simulink model "CDPR_INVERSKINEMATIKK_14_09_23"  (R2022b)
settings: Solver=FixedStepAuto  StartTime=0.0  StopTime=10.0  FixedStep=h  RelTol=1e-3
values from neighbouring files (symbols this model uses):
  a1 = A1 - origin    [CDPR_2R_test.m]    (also in CDPR_2T.m; TEST_INVERSKINEMATIKK.m = [0;1])
  a2 = A2 - origin    [CDPR_2R_test.m]    (also in CDPR_2T.m; TEST_INVERSKINEMATIKK.m = [1;1])
  a3 = A3 - origin    [CDPR_2R_test.m]    (also in CDPR_2T.m; TEST_INVERSKINEMATIKK.m = [0;0])
  a4 = A4 - origin    [CDPR_2R_test.m]    (also in CDPR_2T.m; TEST_INVERSKINEMATIKK.m = [1;0])
  b1 = B1 - body_origin    [CDPR_2R_test.m]    (also in CDPR_2T.m; TEST_INVERSKINEMATIKK.m = [0;L_end/2])
  b2 = B2 - body_origin    [CDPR_2R_test.m]    (also in CDPR_2T.m; TEST_INVERSKINEMATIKK.m = [0;-L_end/2])
  p = [0.5;0.5]    [TEST_INVERSKINEMATIKK.m]
settings Model: Creator=magag  LastModifiedBy=magngrot

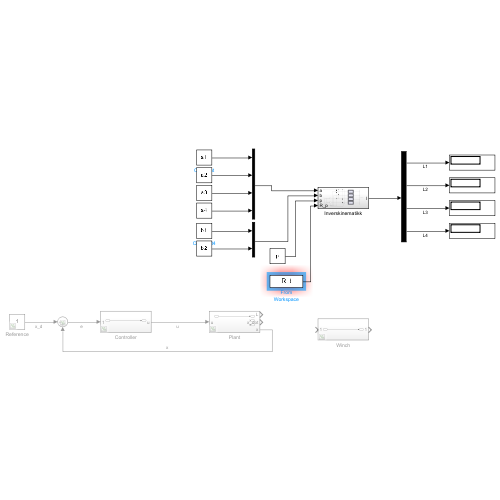
[thumbnail: Simulink's stored preview of the top-level diagram]
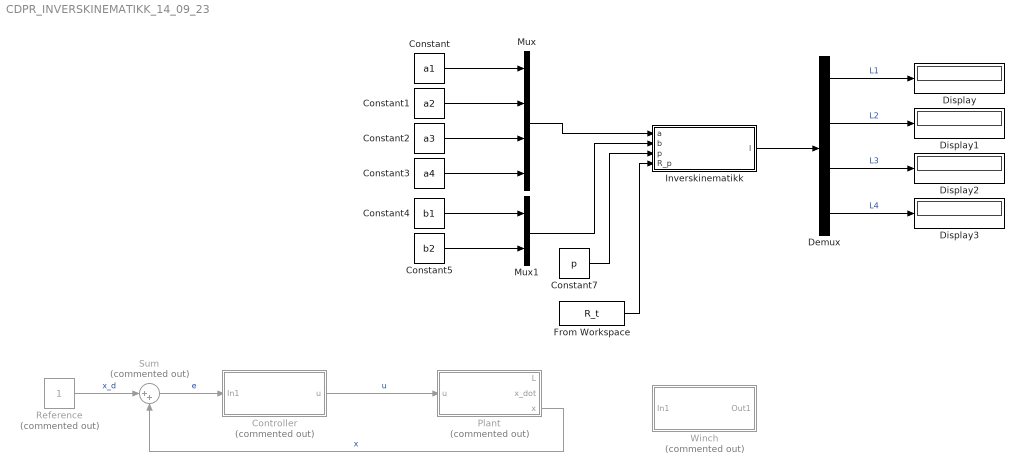
== system CDPR_INVERSKINEMATIKK_14_09_23 ==
  Constant : Constant  Value=a1
  Constant1 : Constant  Value=a2
  Constant2 : Constant  Value=a3
  Constant3 : Constant  Value=a4
  Constant4 : Constant  Value=b1
  Constant5 : Constant  Value=b2
  Constant7 : Constant  Value=p
  Controller : Subsystem  Commented=on
  Demux : Demux
  Display{,1..3} (4 alike) : Display
  From Workspace : FromWorkspace  VariableName=R_t
  Inverskinematikk : Subsystem
  Mux : Mux
  Mux1 : Mux  Inputs=2
  Plant : Subsystem  Commented=on
  Reference : Constant  Commented=on
  Sum : Sum  Commented=on  Inputs=|++
  Winch : Subsystem  Commented=on
  wires:
  Controller/1(u) -> Plant/1(u)  "u"
  Plant/3(x) -> Sum/2  "x"
  Reference/1 -> Sum/1  "x_d"
  Sum/1 -> Controller/1(In1)  "e"
  Constant/1 -> Mux/1
  Constant1/1 -> Mux/2
  Constant2/1 -> Mux/3
  Constant3/1 -> Mux/4
  Mux/1 -> Inverskinematikk/1(a)
  Constant4/1 -> Mux1/1
  Constant5/1 -> Mux1/2
  Mux1/1 -> Inverskinematikk/2(b)
  Inverskinematikk/1(l) -> Demux/1
  Demux/1 -> Display/1  "L1"
  Demux/2 -> Display1/1  "L2"
  Demux/3 -> Display2/1  "L3"
  Demux/4 -> Display3/1  "L4"
  From Workspace/1 -> Inverskinematikk/4(R_p)
  Constant7/1 -> Inverskinematikk/3(p)

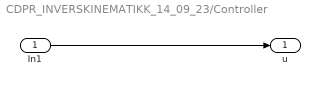
== system CDPR_INVERSKINEMATIKK_14_09_23/Controller ==
  In1 : Inport
  u : Outport
  wires:
  In1/1 -> u/1

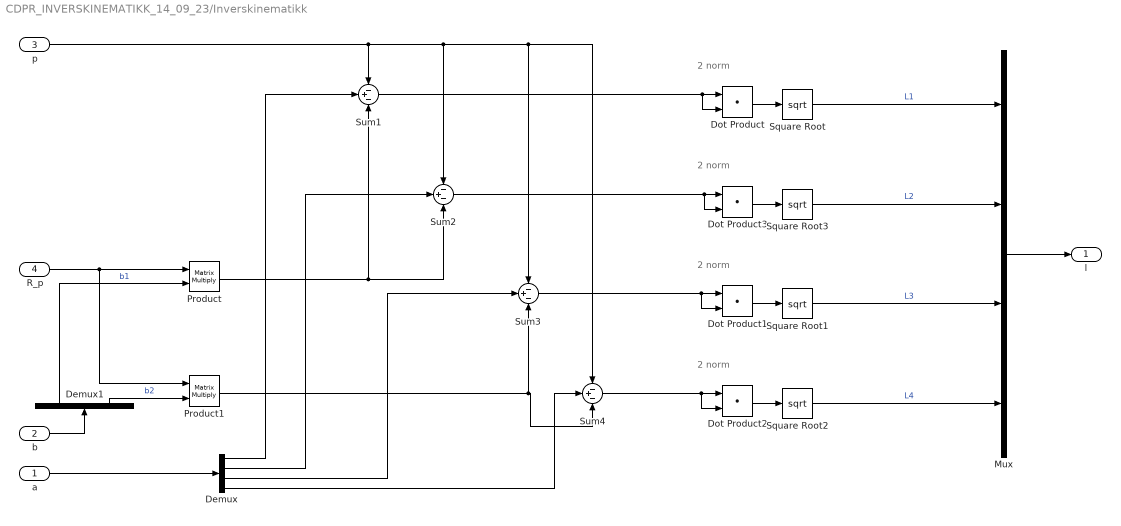
== system CDPR_INVERSKINEMATIKK_14_09_23/Inverskinematikk ==
  note: 2 norm
  note: 2 norm
  note: 2 norm
  note: 2 norm
  a : Inport
  b : Inport  Port=2
  p : Inport  Port=3
  R_p : Inport  Port=4
  Demux : Demux
  Demux1 : Demux  Outputs=2
  Dot Product{,1..3} (4 alike) : DotProduct  OutDataTypeStr=Inherit: Inherit via internal rule
  Mux : Mux
  Product : Product  Multiplication=Matrix(*)
  Product1 : Product  Multiplication=Matrix(*)
  Square Root{,1..3} (4 alike) : Sqrt
  Sum{1..4} (4 alike) : Sum  Inputs=-+-
  l : Outport
  wires:
  R_p/1 -> Product/1, Product1/1
  Dot Product/1 -> Square Root/1
  a/1 -> Demux/1
  b/1 -> Demux1/1
  Dot Product1/1 -> Square Root1/1
  Dot Product2/1 -> Square Root2/1
  Dot Product3/1 -> Square Root3/1
  Demux1/2 -> Product1/2  "b2"
  Demux1/1 -> Product/2  "b1"
  p/1 -> Sum3/1, Sum4/1, Sum2/1, Sum1/1
  Mux/1 -> l/1
  Demux/1 -> Sum1/2
  Demux/2 -> Sum2/2
  Demux/3 -> Sum3/2
  Demux/4 -> Sum4/2
  Product/1 -> Sum2/3, Sum1/3
  Product1/1 -> Sum3/3, Sum4/3
  Sum1/1 -> Dot Product/2, Dot Product/1
  Sum2/1 -> Dot Product3/2, Dot Product3/1
  Sum3/1 -> Dot Product1/2, Dot Product1/1
  Sum4/1 -> Dot Product2/2, Dot Product2/1
  Square Root/1 -> Mux/1  "L1"
  Square Root3/1 -> Mux/2  "L2"
  Square Root1/1 -> Mux/3  "L3"
  Square Root2/1 -> Mux/4  "L4"

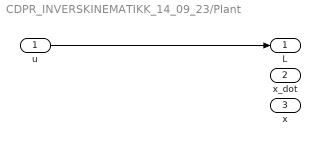
== system CDPR_INVERSKINEMATIKK_14_09_23/Plant ==
  u : Inport
  L : Outport
  x_dot : Outport  Port=2
  x : Outport  Port=3
  wires:
  u/1 -> L/1

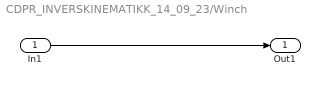
== system CDPR_INVERSKINEMATIKK_14_09_23/Winch ==
  In1 : Inport
  Out1 : Outport
  wires:
  In1/1 -> Out1/1
